simulink model "DriveTrainModel"  (R2025a)
settings: Solver=VariableStepAuto  StartTime=0.0  StopTime=10.0  FixedStep=0.01  RelTol=1e-3
undefined symbols (not defined in the file): L, R
settings Model: DataDictionary=Constants.sldd  Creator=levirogalla  LastModifiedBy=levirogalla

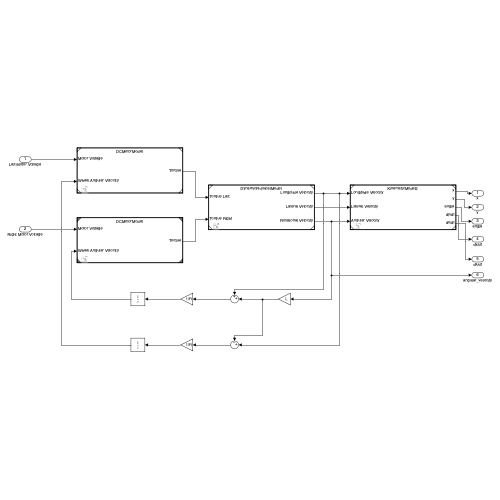
[thumbnail: Simulink's stored preview of the top-level diagram]
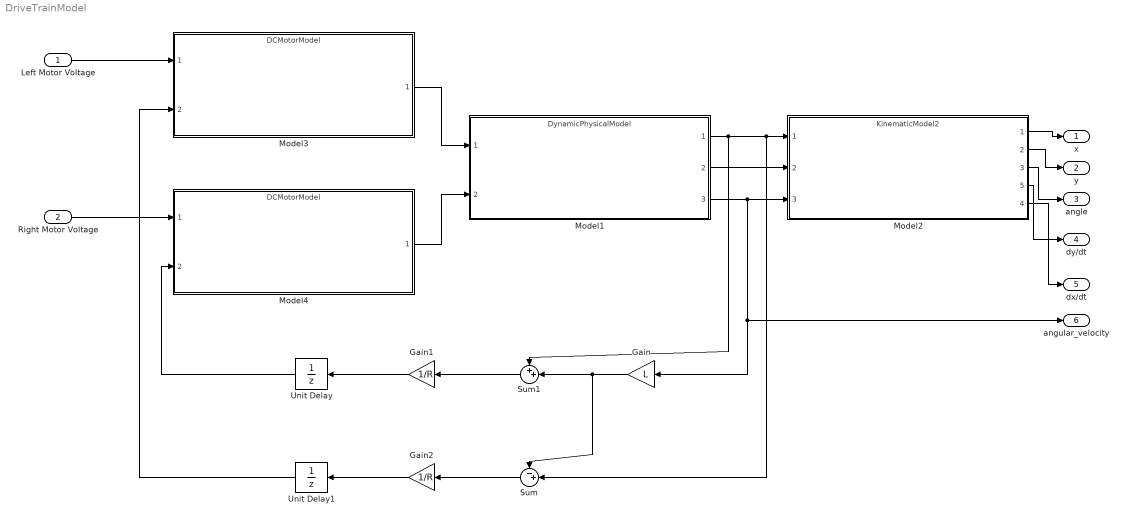
== system DriveTrainModel ==
  Left Motor Voltage : Inport
  Right Motor Voltage : Inport  Port=2
  Gain : Gain  Gain=L
  Gain1 : Gain  Gain=1/R
  Gain2 : Gain  Gain=1/R
  Model1 : ModelReference  ModelNameDialog=DynamicPhysicalModel.slx  SimulationMode=Normal  ModelReferenceVersion=3.1
  Model2 : ModelReference  ModelNameDialog=KinematicModel2.slx  SimulationMode=Normal  ModelReferenceVersion=3.2
      settings: PortSchema="{\"entries\":[{\"content\":{\"sides\":[{\"content\":{\"connectorIds\":[\"In1\",\"In2\",\"In3\"]},\"type\":\"ConnectorPlacement.EquallySpacedRectSide\",\"uuid\":\"40e04a13-7a28-418a-9369-3121e9e226aa\"},{\"content\":{\"connectorIds\":[\"Out1\",\"Out2\",\"Out3\",\"Out5\",\"Out4\"],\"side\":\"RIGHT\"},\"type\":\"ConnectorPlacement.EquallySpacedRectSide\",\"uuid\":\"cc1bc98a-6aae-4b07-b02a-e9b2983d00de\"},{\"content\":{\"side\":\"TOP\"},\"type\":\"ConnectorPlacement.EquallySpacedRectSide\",\"uuid\":\"2247d95d-e44b-4668-885d-ef826e2ae519\"}]},\"type\":\"ConnectorPlacement.EquallySpacedConnector\",\"uuid\":\"0e9473c0-b37b-4274-90f9-c3fd9995d50f\"}],\"packageUris\":[\"http://schema.mathworks.com/mf0/Connector/R2020b\"],\"version\":\"1.0\"}"
  Model3 : ModelReference  ModelNameDialog=DCMotorModel.slx  SimulationMode=Normal  ModelReferenceVersion=3.1
  Model4 : ModelReference  ModelNameDialog=DCMotorModel.slx  SimulationMode=Normal  ModelReferenceVersion=3.1
  Sum : Sum  Inputs=-+|
  Sum1 : Sum  Inputs=++|
  Unit Delay : UnitDelay  SampleTime=-1  HasFrameUpgradeWarning=on
  Unit Delay1 : UnitDelay  SampleTime=-1  HasFrameUpgradeWarning=on
  x : Outport
  y : Outport  Port=2
  angle : Outport  Port=3
  dy/dt : Outport  Port=4
  dx/dt : Outport  Port=5
  angular_velocity : Outport  Port=6
  wires:
  Model1/3 -> Gain/1, angular_velocity/1, Model2/3
  Sum/1 -> Gain2/1
  Gain/1 -> Sum/1, Sum1/2
  Model1/1 -> Sum1/1, Sum/2, Model2/1
  Model3/1 -> Model1/1
  Sum1/1 -> Gain1/1
  Model1/2 -> Model2/2
  Model4/1 -> Model1/2
  Left Motor Voltage/1 -> Model3/1
  Right Motor Voltage/1 -> Model4/1
  Model2/1 -> x/1
  Model2/2 -> y/1
  Model2/3 -> angle/1
  Gain1/1 -> Unit Delay/1
  Gain2/1 -> Unit Delay1/1
  Unit Delay/1 -> Model4/2
  Unit Delay1/1 -> Model3/2
  Model2/5 -> dy/dt/1
  Model2/4 -> dx/dt/1
